simulink library "calcAoA_Beta_relativeSpeed_ul"  (R2020a)
settings: Solver=VariableStepAuto  StartTime=0.0  StopTime=10.0  RelTol=1e-3
libraries: calcVectorMagnitude_ul x1
settings Model: Creator=Ayaz  LastModifiedBy=Ayaz

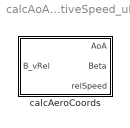
== system calcAoA_Beta_relativeSpeed_ul ==
  calcAeroCoords : Subsystem

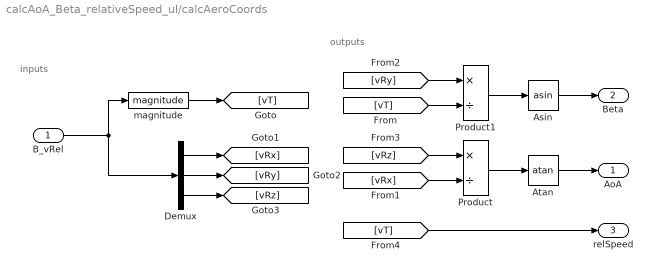
== system calcAoA_Beta_relativeSpeed_ul/calcAeroCoords ==
  note: outputs
  note: inputs
  B_vRel : Inport
  Asin : Trigonometry  Operator=asin
  Atan : Trigonometry  Operator=atan
  Demux : Demux  Outputs=3
  Product : Product  Inputs=*/
  Product1 : Product  Inputs=*/
  magnitude : calcVectorMagnitude_ul/magnitude  SystemSampleTime=-1  Latency=0  AutoFrameSizeCalculation=off
  AoA : Outport
  Beta : Outport  Port=2
  relSpeed : Outport  Port=3
  wires:
  B_vRel/1 -> Demux/1, magnitude/1
  Demux/1 -> [vRx]
  Demux/2 -> [vRy]
  Demux/3 -> [vRz]
  magnitude/1 -> [vT]
  [vRz] -> Product/1
  [vRx] -> Product/2
  Product/1 -> Atan/1
  [vRy] -> Product1/1
  [vT] -> Product1/2
  Asin/1 -> Beta/1
  Product1/1 -> Asin/1
  Atan/1 -> AoA/1
  [vT] -> relSpeed/1
